simulink model "SimForces2020a"  (R2020a)
settings: Solver=daessc  StartTime=0.0  StopTime=10  FixedStep=0.001  RelTol=1e-4
values from neighbouring files (symbols this model uses):
  Bc1_V = [0;0;0;0;0;0]    [initializeSimulationGP.m]
  D22F = [0;0;0;0;0;0]    [initializeSimulationGP.m]
  filtDV = init2ndOrderLowPassFilter(35*2*pi,1,controller.dT)    [initializeLowPassFilters.m]
  filtEnc = init2ndOrderLowPassFilter(35*2*pi,1,controller.dT)    [initializeLowPassFilters.m]
undefined symbols (not defined in the file or in its folder): aux, B11_r_B11Tc1, B11_V, B11Ftot, B12_r_B12Tc2, B12_Rot_Tc2, B12_U_Tc2, B12_V, B12Ftot, B31_r_B31B41, B31_V, B31FTot, B32_r_B32B42, B32_Rot_B42, B32_U_B42, B32_V, B32FTot, B41_r_B41Tc1, B41_V, B41FTot, B42_r_B42Tc2, B42_Rot_Tc2, B42_U_Tc2, B42_V, B42FTot, B52_r_B52P32, B52_Rot_P32, B52_U_P32, B52_V, B52Ftot, Bc1_r_Bc1B11, Bc1_r_Bc1B31, Bc1FTot, Bc2_r_Bc2B12, Bc2_r_Bc2B32, Bc2_Rot_B12, Bc2_Rot_B32, Bc2_U_B12, Bc2_U_B32, Bc2_V, Bc2Tot, cmdMotion, controller, cyl1, cyl2, D22_V, dq1, dq11, dq12, dq2, dq21, dq22, dx1, dx2, dxt2, fc1, fc1r, fc2, fc2r, fct2 ... (+62)
libraries: sm_lib x31, nesl_utility x10
(part 5 of 7)

== system SimForces2020a/sbVDCController/sbFormTotalRequiredForces/sbTotalRequiredForcesPS2/sbFilteredVelocityDerivativeP32/sbLowPassFilter4 ==
  dV : Inport
  Delay : Delay  InitialConditionSource=Input port  SampleTime=filtDV.dT
      settings: InputPortMap=u0,p4
  Delay1 : Delay  DelayLength=1  InitialConditionSource=Input port  SampleTime=filtDV.dT
      settings: InputPortMap=u0,p4
  Delay2 : Delay  DelayLength=0  InitialConditionSource=Input port  SampleTime=filtDV.dT
      settings: InputPortMap=u0,p4
  Delay3 : Delay  InitialConditionSource=Input port  SampleTime=filtDV.dT
      settings: InputPortMap=u0,p4
  Delay4 : Delay  DelayLength=1  InitialConditionSource=Input port  SampleTime=filtDV.dT
      settings: InputPortMap=u0,p4
  Gain : Gain  Gain=filtDV.a0
  Gain1 : Gain  Gain=filtDV.b1
  Gain2 : Gain  Gain=filtDV.b2
  Gain3 : Gain  Gain=filtDV.b0
  Gain4 : Gain  Gain=filtDV.a1
  Sum : Sum  Inputs=|--+++
  dVFilt : Outport
  wires:
  Delay3/1 -> Gain3/1
  Gain/1 -> Sum/2
  Gain1/1 -> Sum/4
  dV/1 -> Delay/2, Delay4/2, Delay1/2, Delay3/1, Delay3/2, Delay1/1, Delay2/2, Delay2/1  "dV"
  Sum/1 -> Delay/1, Delay4/1, dVFilt/1  "dVFilt"
  Gain4/1 -> Sum/1
  Delay2/1 -> Gain2/1
  Delay1/1 -> Gain1/1
  Delay/1 -> Gain/1
  Delay4/1 -> Gain4/1
  Gain2/1 -> Sum/3
  Gain3/1 -> Sum/5

== system SimForces2020a/sbVDCController/sbFormTotalRequiredForces/sbTotalRequiredForcesPS2/sbFilteredVelocityDerivativeP32/sbLowPassFilter5 ==
  dV : Inport
  Delay : Delay  InitialConditionSource=Input port  SampleTime=filtDV.dT
      settings: InputPortMap=u0,p4
  Delay1 : Delay  DelayLength=1  InitialConditionSource=Input port  SampleTime=filtDV.dT
      settings: InputPortMap=u0,p4
  Delay2 : Delay  DelayLength=0  InitialConditionSource=Input port  SampleTime=filtDV.dT
      settings: InputPortMap=u0,p4
  Delay3 : Delay  InitialConditionSource=Input port  SampleTime=filtDV.dT
      settings: InputPortMap=u0,p4
  Delay4 : Delay  DelayLength=1  InitialConditionSource=Input port  SampleTime=filtDV.dT
      settings: InputPortMap=u0,p4
  Gain : Gain  Gain=filtDV.a0
  Gain1 : Gain  Gain=filtDV.b1
  Gain2 : Gain  Gain=filtDV.b2
  Gain3 : Gain  Gain=filtDV.b0
  Gain4 : Gain  Gain=filtDV.a1
  Sum : Sum  Inputs=|--+++
  dVFilt : Outport
  wires:
  Gain3/1 -> Sum/5
  Gain2/1 -> Sum/3
  Delay4/1 -> Gain4/1
  Delay/1 -> Gain/1
  Delay1/1 -> Gain1/1
  Delay2/1 -> Gain2/1
  Gain4/1 -> Sum/1
  Sum/1 -> dVFilt/1, Delay4/1, Delay/1  "dVFilt"
  dV/1 -> Delay2/1, Delay2/2, Delay1/1, Delay3/2, Delay3/1, Delay1/2, Delay4/2, Delay/2  "dV"
  Gain1/1 -> Sum/4
  Gain/1 -> Sum/2
  Delay3/1 -> Gain3/1

== system SimForces2020a/sbVDCController/sbFormTotalRequiredForces/sbTotalRequiredForcesPS2/sbFilteredVelocityDerivativeP32/sbLowPassFilter6 ==
  dV : Inport
  Delay : Delay  InitialConditionSource=Input port  SampleTime=filtDV.dT
      settings: InputPortMap=u0,p4
  Delay1 : Delay  DelayLength=1  InitialConditionSource=Input port  SampleTime=filtDV.dT
      settings: InputPortMap=u0,p4
  Delay2 : Delay  DelayLength=0  InitialConditionSource=Input port  SampleTime=filtDV.dT
      settings: InputPortMap=u0,p4
  Delay3 : Delay  InitialConditionSource=Input port  SampleTime=filtDV.dT
      settings: InputPortMap=u0,p4
  Delay4 : Delay  DelayLength=1  InitialConditionSource=Input port  SampleTime=filtDV.dT
      settings: InputPortMap=u0,p4
  Gain : Gain  Gain=filtDV.a0
  Gain1 : Gain  Gain=filtDV.b1
  Gain2 : Gain  Gain=filtDV.b2
  Gain3 : Gain  Gain=filtDV.b0
  Gain4 : Gain  Gain=filtDV.a1
  Sum : Sum  Inputs=|--+++
  dVFilt : Outport
  wires:
  Delay3/1 -> Gain3/1
  Gain/1 -> Sum/2
  Gain1/1 -> Sum/4
  dV/1 -> Delay/2, Delay4/2, Delay1/2, Delay3/1, Delay3/2, Delay1/1, Delay2/2, Delay2/1  "dV"
  Sum/1 -> Delay/1, Delay4/1, dVFilt/1  "dVFilt"
  Gain4/1 -> Sum/1
  Delay2/1 -> Gain2/1
  Delay1/1 -> Gain1/1
  Delay/1 -> Gain/1
  Delay4/1 -> Gain4/1
  Gain2/1 -> Sum/3
  Gain3/1 -> Sum/5

== system SimForces2020a/sbVDCController/sbFormTotalRequiredForces/sbTotalRequiredForcesRS1/sbFilteredVelocityDerivativeB11/sbDiscreteDerivative1 ==
  u : Inport
  Add : Sum  Inputs=-+
  Gain6 : Gain  Gain=1/(2*controller.dT)
  Integer Delay : Delay  InitialConditionSource=Input port  InitialCondition=0  SampleTime=controller.dT
      settings: InputPortMap=u0,p4
  du/dt : Outport  PortDimensions=1
  wires:
  Gain6/1 -> du/dt/1
  Integer Delay/1 -> Add/1
  u/1 -> Add/2, Integer Delay/2, Integer Delay/1
  Add/1 -> Gain6/1

== system SimForces2020a/sbVDCController/sbFormTotalRequiredForces/sbTotalRequiredForcesRS1/sbFilteredVelocityDerivativeB11/sbDiscreteDerivative2 ==
  u : Inport
  Add : Sum  Inputs=-+
  Gain6 : Gain  Gain=1/(2*controller.dT)
  Integer Delay : Delay  InitialConditionSource=Input port  InitialCondition=0  SampleTime=controller.dT
      settings: InputPortMap=u0,p4
  du/dt : Outport  PortDimensions=1
  wires:
  Gain6/1 -> du/dt/1
  Add/1 -> Gain6/1
  Integer Delay/1 -> Add/1
  u/1 -> Add/2, Integer Delay/2, Integer Delay/1

== system SimForces2020a/sbVDCController/sbFormTotalRequiredForces/sbTotalRequiredForcesRS1/sbFilteredVelocityDerivativeB11/sbDiscreteDerivative3 ==
  u : Inport
  Add : Sum  Inputs=-+
  Gain6 : Gain  Gain=1/(2*controller.dT)
  Integer Delay : Delay  InitialConditionSource=Input port  InitialCondition=0  SampleTime=controller.dT
      settings: InputPortMap=u0,p4
  du/dt : Outport  PortDimensions=1
  wires:
  Gain6/1 -> du/dt/1
  u/1 -> Add/2, Integer Delay/2, Integer Delay/1
  Integer Delay/1 -> Add/1
  Add/1 -> Gain6/1

== system SimForces2020a/sbVDCController/sbFormTotalRequiredForces/sbTotalRequiredForcesRS1/sbFilteredVelocityDerivativeB11/sbDiscreteDerivative4 ==
  u : Inport
  Add : Sum  Inputs=-+
  Gain6 : Gain  Gain=1/(2*controller.dT)
  Integer Delay : Delay  InitialConditionSource=Input port  InitialCondition=0  SampleTime=controller.dT
      settings: InputPortMap=u0,p4
  du/dt : Outport  PortDimensions=1
  wires:
  Gain6/1 -> du/dt/1
  u/1 -> Add/2, Integer Delay/2, Integer Delay/1
  Integer Delay/1 -> Add/1
  Add/1 -> Gain6/1

== system SimForces2020a/sbVDCController/sbFormTotalRequiredForces/sbTotalRequiredForcesRS1/sbFilteredVelocityDerivativeB11/sbDiscreteDerivative5 ==
  u : Inport
  Add : Sum  Inputs=-+
  Gain6 : Gain  Gain=1/(2*controller.dT)
  Integer Delay : Delay  InitialConditionSource=Input port  InitialCondition=0  SampleTime=controller.dT
      settings: InputPortMap=u0,p4
  du/dt : Outport  PortDimensions=1
  wires:
  Gain6/1 -> du/dt/1
  u/1 -> Add/2, Integer Delay/2, Integer Delay/1
  Integer Delay/1 -> Add/1
  Add/1 -> Gain6/1

== system SimForces2020a/sbVDCController/sbFormTotalRequiredForces/sbTotalRequiredForcesRS1/sbFilteredVelocityDerivativeB11/sbDiscreteDerivative6 ==
  u : Inport
  Add : Sum  Inputs=-+
  Gain6 : Gain  Gain=1/(2*controller.dT)
  Integer Delay : Delay  InitialConditionSource=Input port  InitialCondition=0  SampleTime=controller.dT
      settings: InputPortMap=u0,p4
  du/dt : Outport  PortDimensions=1
  wires:
  Gain6/1 -> du/dt/1
  u/1 -> Add/2, Integer Delay/2, Integer Delay/1
  Integer Delay/1 -> Add/1
  Add/1 -> Gain6/1

== system SimForces2020a/sbVDCController/sbFormTotalRequiredForces/sbTotalRequiredForcesRS1/sbFilteredVelocityDerivativeB11/sbLowPassFilter1 ==
  dV : Inport
  Delay : Delay  InitialConditionSource=Input port  SampleTime=filtDV.dT
      settings: InputPortMap=u0,p4
  Delay1 : Delay  DelayLength=1  InitialConditionSource=Input port  SampleTime=filtDV.dT
      settings: InputPortMap=u0,p4
  Delay2 : Delay  DelayLength=0  InitialConditionSource=Input port  SampleTime=filtDV.dT
      settings: InputPortMap=u0,p4
  Delay3 : Delay  InitialConditionSource=Input port  SampleTime=filtDV.dT
      settings: InputPortMap=u0,p4
  Delay4 : Delay  DelayLength=1  InitialConditionSource=Input port  SampleTime=filtDV.dT
      settings: InputPortMap=u0,p4
  Gain : Gain  Gain=filtDV.a0
  Gain1 : Gain  Gain=filtDV.b1
  Gain2 : Gain  Gain=filtDV.b2
  Gain3 : Gain  Gain=filtDV.b0
  Gain4 : Gain  Gain=filtDV.a1
  Sum : Sum  Inputs=|--+++
  dVFilt : Outport
  wires:
  Delay3/1 -> Gain3/1
  Gain/1 -> Sum/2
  Gain1/1 -> Sum/4
  dV/1 -> Delay/2, Delay4/2, Delay1/2, Delay3/1, Delay3/2, Delay1/1, Delay2/2, Delay2/1  "dV"
  Sum/1 -> Delay/1, Delay4/1, dVFilt/1  "dVFilt"
  Gain4/1 -> Sum/1
  Delay2/1 -> Gain2/1
  Delay1/1 -> Gain1/1
  Delay/1 -> Gain/1
  Delay4/1 -> Gain4/1
  Gain2/1 -> Sum/3
  Gain3/1 -> Sum/5

== system SimForces2020a/sbVDCController/sbFormTotalRequiredForces/sbTotalRequiredForcesRS1/sbFilteredVelocityDerivativeB11/sbLowPassFilter2 ==
  dV : Inport
  Delay : Delay  InitialConditionSource=Input port  SampleTime=filtDV.dT
      settings: InputPortMap=u0,p4
  Delay1 : Delay  DelayLength=1  InitialConditionSource=Input port  SampleTime=filtDV.dT
      settings: InputPortMap=u0,p4
  Delay2 : Delay  DelayLength=0  InitialConditionSource=Input port  SampleTime=filtDV.dT
      settings: InputPortMap=u0,p4
  Delay3 : Delay  InitialConditionSource=Input port  SampleTime=filtDV.dT
      settings: InputPortMap=u0,p4
  Delay4 : Delay  DelayLength=1  InitialConditionSource=Input port  SampleTime=filtDV.dT
      settings: InputPortMap=u0,p4
  Gain : Gain  Gain=filtDV.a0
  Gain1 : Gain  Gain=filtDV.b1
  Gain2 : Gain  Gain=filtDV.b2
  Gain3 : Gain  Gain=filtDV.b0
  Gain4 : Gain  Gain=filtDV.a1
  Sum : Sum  Inputs=|--+++
  dVFilt : Outport
  wires:
  Gain3/1 -> Sum/5
  Gain2/1 -> Sum/3
  Delay4/1 -> Gain4/1
  Delay/1 -> Gain/1
  Delay1/1 -> Gain1/1
  Delay2/1 -> Gain2/1
  Gain4/1 -> Sum/1
  Sum/1 -> dVFilt/1, Delay4/1, Delay/1  "dVFilt"
  dV/1 -> Delay2/1, Delay2/2, Delay1/1, Delay3/2, Delay3/1, Delay1/2, Delay4/2, Delay/2  "dV"
  Gain1/1 -> Sum/4
  Gain/1 -> Sum/2
  Delay3/1 -> Gain3/1

== system SimForces2020a/sbVDCController/sbFormTotalRequiredForces/sbTotalRequiredForcesRS1/sbFilteredVelocityDerivativeB11/sbLowPassFilter3 ==
  dV : Inport
  Delay : Delay  InitialConditionSource=Input port  SampleTime=filtDV.dT
      settings: InputPortMap=u0,p4
  Delay1 : Delay  DelayLength=1  InitialConditionSource=Input port  SampleTime=filtDV.dT
      settings: InputPortMap=u0,p4
  Delay2 : Delay  DelayLength=0  InitialConditionSource=Input port  SampleTime=filtDV.dT
      settings: InputPortMap=u0,p4
  Delay3 : Delay  InitialConditionSource=Input port  SampleTime=filtDV.dT
      settings: InputPortMap=u0,p4
  Delay4 : Delay  DelayLength=1  InitialConditionSource=Input port  SampleTime=filtDV.dT
      settings: InputPortMap=u0,p4
  Gain : Gain  Gain=filtDV.a0
  Gain1 : Gain  Gain=filtDV.b1
  Gain2 : Gain  Gain=filtDV.b2
  Gain3 : Gain  Gain=filtDV.b0
  Gain4 : Gain  Gain=filtDV.a1
  Sum : Sum  Inputs=|--+++
  dVFilt : Outport
  wires:
  Delay3/1 -> Gain3/1
  Gain/1 -> Sum/2
  Gain1/1 -> Sum/4
  dV/1 -> Delay/2, Delay4/2, Delay1/2, Delay3/1, Delay3/2, Delay1/1, Delay2/2, Delay2/1  "dV"
  Sum/1 -> Delay/1, Delay4/1, dVFilt/1  "dVFilt"
  Gain4/1 -> Sum/1
  Delay2/1 -> Gain2/1
  Delay1/1 -> Gain1/1
  Delay/1 -> Gain/1
  Delay4/1 -> Gain4/1
  Gain2/1 -> Sum/3
  Gain3/1 -> Sum/5

== system SimForces2020a/sbVDCController/sbFormTotalRequiredForces/sbTotalRequiredForcesRS1/sbFilteredVelocityDerivativeB11/sbLowPassFilter4 ==
  dV : Inport
  Delay : Delay  InitialConditionSource=Input port  SampleTime=filtDV.dT
      settings: InputPortMap=u0,p4
  Delay1 : Delay  DelayLength=1  InitialConditionSource=Input port  SampleTime=filtDV.dT
      settings: InputPortMap=u0,p4
  Delay2 : Delay  DelayLength=0  InitialConditionSource=Input port  SampleTime=filtDV.dT
      settings: InputPortMap=u0,p4
  Delay3 : Delay  InitialConditionSource=Input port  SampleTime=filtDV.dT
      settings: InputPortMap=u0,p4
  Delay4 : Delay  DelayLength=1  InitialConditionSource=Input port  SampleTime=filtDV.dT
      settings: InputPortMap=u0,p4
  Gain : Gain  Gain=filtDV.a0
  Gain1 : Gain  Gain=filtDV.b1
  Gain2 : Gain  Gain=filtDV.b2
  Gain3 : Gain  Gain=filtDV.b0
  Gain4 : Gain  Gain=filtDV.a1
  Sum : Sum  Inputs=|--+++
  dVFilt : Outport
  wires:
  Gain3/1 -> Sum/5
  Gain2/1 -> Sum/3
  Delay4/1 -> Gain4/1
  Delay/1 -> Gain/1
  Delay1/1 -> Gain1/1
  Delay2/1 -> Gain2/1
  Gain4/1 -> Sum/1
  Sum/1 -> dVFilt/1, Delay4/1, Delay/1  "dVFilt"
  dV/1 -> Delay2/1, Delay2/2, Delay1/1, Delay3/2, Delay3/1, Delay1/2, Delay4/2, Delay/2  "dV"
  Gain1/1 -> Sum/4
  Gain/1 -> Sum/2
  Delay3/1 -> Gain3/1

== system SimForces2020a/sbVDCController/sbFormTotalRequiredForces/sbTotalRequiredForcesRS1/sbFilteredVelocityDerivativeB11/sbLowPassFilter5 ==
  dV : Inport
  Delay : Delay  InitialConditionSource=Input port  SampleTime=filtDV.dT
      settings: InputPortMap=u0,p4
  Delay1 : Delay  DelayLength=1  InitialConditionSource=Input port  SampleTime=filtDV.dT
      settings: InputPortMap=u0,p4
  Delay2 : Delay  DelayLength=0  InitialConditionSource=Input port  SampleTime=filtDV.dT
      settings: InputPortMap=u0,p4
  Delay3 : Delay  InitialConditionSource=Input port  SampleTime=filtDV.dT
      settings: InputPortMap=u0,p4
  Delay4 : Delay  DelayLength=1  InitialConditionSource=Input port  SampleTime=filtDV.dT
      settings: InputPortMap=u0,p4
  Gain : Gain  Gain=filtDV.a0
  Gain1 : Gain  Gain=filtDV.b1
  Gain2 : Gain  Gain=filtDV.b2
  Gain3 : Gain  Gain=filtDV.b0
  Gain4 : Gain  Gain=filtDV.a1
  Sum : Sum  Inputs=|--+++
  dVFilt : Outport
  wires:
  Delay3/1 -> Gain3/1
  Gain/1 -> Sum/2
  Gain1/1 -> Sum/4
  dV/1 -> Delay/2, Delay4/2, Delay1/2, Delay3/1, Delay3/2, Delay1/1, Delay2/2, Delay2/1  "dV"
  Sum/1 -> Delay/1, Delay4/1, dVFilt/1  "dVFilt"
  Gain4/1 -> Sum/1
  Delay2/1 -> Gain2/1
  Delay1/1 -> Gain1/1
  Delay/1 -> Gain/1
  Delay4/1 -> Gain4/1
  Gain2/1 -> Sum/3
  Gain3/1 -> Sum/5

== system SimForces2020a/sbVDCController/sbFormTotalRequiredForces/sbTotalRequiredForcesRS1/sbFilteredVelocityDerivativeB11/sbLowPassFilter6 ==
  dV : Inport
  Delay : Delay  InitialConditionSource=Input port  SampleTime=filtDV.dT
      settings: InputPortMap=u0,p4
  Delay1 : Delay  DelayLength=1  InitialConditionSource=Input port  SampleTime=filtDV.dT
      settings: InputPortMap=u0,p4
  Delay2 : Delay  DelayLength=0  InitialConditionSource=Input port  SampleTime=filtDV.dT
      settings: InputPortMap=u0,p4
  Delay3 : Delay  InitialConditionSource=Input port  SampleTime=filtDV.dT
      settings: InputPortMap=u0,p4
  Delay4 : Delay  DelayLength=1  InitialConditionSource=Input port  SampleTime=filtDV.dT
      settings: InputPortMap=u0,p4
  Gain : Gain  Gain=filtDV.a0
  Gain1 : Gain  Gain=filtDV.b1
  Gain2 : Gain  Gain=filtDV.b2
  Gain3 : Gain  Gain=filtDV.b0
  Gain4 : Gain  Gain=filtDV.a1
  Sum : Sum  Inputs=|--+++
  dVFilt : Outport
  wires:
  Gain3/1 -> Sum/5
  Gain2/1 -> Sum/3
  Delay4/1 -> Gain4/1
  Delay/1 -> Gain/1
  Delay1/1 -> Gain1/1
  Delay2/1 -> Gain2/1
  Gain4/1 -> Sum/1
  Sum/1 -> dVFilt/1, Delay4/1, Delay/1  "dVFilt"
  dV/1 -> Delay2/1, Delay2/2, Delay1/1, Delay3/2, Delay3/1, Delay1/2, Delay4/2, Delay/2  "dV"
  Gain1/1 -> Sum/4
  Gain/1 -> Sum/2
  Delay3/1 -> Gain3/1

== system SimForces2020a/sbVDCController/sbFormTotalRequiredForces/sbTotalRequiredForcesRS1/sbFilteredVelocityDerivativeB31/sbDiscreteDerivative1 ==
  u : Inport
  Add : Sum  Inputs=-+
  Gain6 : Gain  Gain=1/(2*controller.dT)
  Integer Delay : Delay  InitialConditionSource=Input port  InitialCondition=0  SampleTime=controller.dT
      settings: InputPortMap=u0,p4
  du/dt : Outport  PortDimensions=1
  wires:
  Add/1 -> Gain6/1
  u/1 -> Integer Delay/1, Integer Delay/2, Add/2
  Integer Delay/1 -> Add/1
  Gain6/1 -> du/dt/1

== system SimForces2020a/sbVDCController/sbFormTotalRequiredForces/sbTotalRequiredForcesRS1/sbFilteredVelocityDerivativeB31/sbDiscreteDerivative2 ==
  u : Inport
  Add : Sum  Inputs=-+
  Gain6 : Gain  Gain=1/(2*controller.dT)
  Integer Delay : Delay  InitialConditionSource=Input port  InitialCondition=0  SampleTime=controller.dT
      settings: InputPortMap=u0,p4
  du/dt : Outport  PortDimensions=1
  wires:
  u/1 -> Integer Delay/1, Integer Delay/2, Add/2
  Integer Delay/1 -> Add/1
  Add/1 -> Gain6/1
  Gain6/1 -> du/dt/1

== system SimForces2020a/sbVDCController/sbFormTotalRequiredForces/sbTotalRequiredForcesRS1/sbFilteredVelocityDerivativeB31/sbDiscreteDerivative3 ==
  u : Inport
  Add : Sum  Inputs=-+
  Gain6 : Gain  Gain=1/(2*controller.dT)
  Integer Delay : Delay  InitialConditionSource=Input port  InitialCondition=0  SampleTime=controller.dT
      settings: InputPortMap=u0,p4
  du/dt : Outport  PortDimensions=1
  wires:
  Add/1 -> Gain6/1
  Integer Delay/1 -> Add/1
  u/1 -> Integer Delay/1, Integer Delay/2, Add/2
  Gain6/1 -> du/dt/1

== system SimForces2020a/sbVDCController/sbFormTotalRequiredForces/sbTotalRequiredForcesRS1/sbFilteredVelocityDerivativeB31/sbDiscreteDerivative4 ==
  u : Inport
  Add : Sum  Inputs=-+
  Gain6 : Gain  Gain=1/(2*controller.dT)
  Integer Delay : Delay  InitialConditionSource=Input port  InitialCondition=0  SampleTime=controller.dT
      settings: InputPortMap=u0,p4
  du/dt : Outport  PortDimensions=1
  wires:
  Add/1 -> Gain6/1
  Integer Delay/1 -> Add/1
  u/1 -> Integer Delay/1, Integer Delay/2, Add/2
  Gain6/1 -> du/dt/1

== system SimForces2020a/sbVDCController/sbFormTotalRequiredForces/sbTotalRequiredForcesRS1/sbFilteredVelocityDerivativeB31/sbDiscreteDerivative5 ==
  u : Inport
  Add : Sum  Inputs=-+
  Gain6 : Gain  Gain=1/(2*controller.dT)
  Integer Delay : Delay  InitialConditionSource=Input port  InitialCondition=0  SampleTime=controller.dT
      settings: InputPortMap=u0,p4
  du/dt : Outport  PortDimensions=1
  wires:
  Add/1 -> Gain6/1
  Integer Delay/1 -> Add/1
  u/1 -> Integer Delay/1, Integer Delay/2, Add/2
  Gain6/1 -> du/dt/1

== system SimForces2020a/sbVDCController/sbFormTotalRequiredForces/sbTotalRequiredForcesRS1/sbFilteredVelocityDerivativeB31/sbDiscreteDerivative6 ==
  u : Inport
  Add : Sum  Inputs=-+
  Gain6 : Gain  Gain=1/(2*controller.dT)
  Integer Delay : Delay  InitialConditionSource=Input port  InitialCondition=0  SampleTime=controller.dT
      settings: InputPortMap=u0,p4
  du/dt : Outport  PortDimensions=1
  wires:
  Add/1 -> Gain6/1
  Integer Delay/1 -> Add/1
  u/1 -> Integer Delay/1, Integer Delay/2, Add/2
  Gain6/1 -> du/dt/1

== system SimForces2020a/sbVDCController/sbFormTotalRequiredForces/sbTotalRequiredForcesRS1/sbFilteredVelocityDerivativeB31/sbLowPassFilter1 ==
  dV : Inport
  Delay : Delay  InitialConditionSource=Input port  SampleTime=filtDV.dT
      settings: InputPortMap=u0,p4
  Delay1 : Delay  DelayLength=1  InitialConditionSource=Input port  SampleTime=filtDV.dT
      settings: InputPortMap=u0,p4
  Delay2 : Delay  DelayLength=0  InitialConditionSource=Input port  SampleTime=filtDV.dT
      settings: InputPortMap=u0,p4
  Delay3 : Delay  InitialConditionSource=Input port  SampleTime=filtDV.dT
      settings: InputPortMap=u0,p4
  Delay4 : Delay  DelayLength=1  InitialConditionSource=Input port  SampleTime=filtDV.dT
      settings: InputPortMap=u0,p4
  Gain : Gain  Gain=filtDV.a0
  Gain1 : Gain  Gain=filtDV.b1
  Gain2 : Gain  Gain=filtDV.b2
  Gain3 : Gain  Gain=filtDV.b0
  Gain4 : Gain  Gain=filtDV.a1
  Sum : Sum  Inputs=|--+++
  dVFilt : Outport
  wires:
  Gain3/1 -> Sum/5
  Gain2/1 -> Sum/3
  Delay4/1 -> Gain4/1
  Delay/1 -> Gain/1
  Delay1/1 -> Gain1/1
  Delay2/1 -> Gain2/1
  Gain4/1 -> Sum/1
  Sum/1 -> dVFilt/1, Delay4/1, Delay/1  "dVFilt"
  dV/1 -> Delay2/1, Delay2/2, Delay1/1, Delay3/2, Delay3/1, Delay1/2, Delay4/2, Delay/2  "dV"
  Gain1/1 -> Sum/4
  Gain/1 -> Sum/2
  Delay3/1 -> Gain3/1

== system SimForces2020a/sbVDCController/sbFormTotalRequiredForces/sbTotalRequiredForcesRS1/sbFilteredVelocityDerivativeB31/sbLowPassFilter2 ==
  dV : Inport
  Delay : Delay  InitialConditionSource=Input port  SampleTime=filtDV.dT
      settings: InputPortMap=u0,p4
  Delay1 : Delay  DelayLength=1  InitialConditionSource=Input port  SampleTime=filtDV.dT
      settings: InputPortMap=u0,p4
  Delay2 : Delay  DelayLength=0  InitialConditionSource=Input port  SampleTime=filtDV.dT
      settings: InputPortMap=u0,p4
  Delay3 : Delay  InitialConditionSource=Input port  SampleTime=filtDV.dT
      settings: InputPortMap=u0,p4
  Delay4 : Delay  DelayLength=1  InitialConditionSource=Input port  SampleTime=filtDV.dT
      settings: InputPortMap=u0,p4
  Gain : Gain  Gain=filtDV.a0
  Gain1 : Gain  Gain=filtDV.b1
  Gain2 : Gain  Gain=filtDV.b2
  Gain3 : Gain  Gain=filtDV.b0
  Gain4 : Gain  Gain=filtDV.a1
  Sum : Sum  Inputs=|--+++
  dVFilt : Outport
  wires:
  Delay3/1 -> Gain3/1
  Gain/1 -> Sum/2
  Gain1/1 -> Sum/4
  dV/1 -> Delay/2, Delay4/2, Delay1/2, Delay3/1, Delay3/2, Delay1/1, Delay2/2, Delay2/1  "dV"
  Sum/1 -> Delay/1, Delay4/1, dVFilt/1  "dVFilt"
  Gain4/1 -> Sum/1
  Delay2/1 -> Gain2/1
  Delay1/1 -> Gain1/1
  Delay/1 -> Gain/1
  Delay4/1 -> Gain4/1
  Gain2/1 -> Sum/3
  Gain3/1 -> Sum/5

== system SimForces2020a/sbVDCController/sbFormTotalRequiredForces/sbTotalRequiredForcesRS1/sbFilteredVelocityDerivativeB31/sbLowPassFilter3 ==
  dV : Inport
  Delay : Delay  InitialConditionSource=Input port  SampleTime=filtDV.dT
      settings: InputPortMap=u0,p4
  Delay1 : Delay  DelayLength=1  InitialConditionSource=Input port  SampleTime=filtDV.dT
      settings: InputPortMap=u0,p4
  Delay2 : Delay  DelayLength=0  InitialConditionSource=Input port  SampleTime=filtDV.dT
      settings: InputPortMap=u0,p4
  Delay3 : Delay  InitialConditionSource=Input port  SampleTime=filtDV.dT
      settings: InputPortMap=u0,p4
  Delay4 : Delay  DelayLength=1  InitialConditionSource=Input port  SampleTime=filtDV.dT
      settings: InputPortMap=u0,p4
  Gain : Gain  Gain=filtDV.a0
  Gain1 : Gain  Gain=filtDV.b1
  Gain2 : Gain  Gain=filtDV.b2
  Gain3 : Gain  Gain=filtDV.b0
  Gain4 : Gain  Gain=filtDV.a1
  Sum : Sum  Inputs=|--+++
  dVFilt : Outport
  wires:
  Gain3/1 -> Sum/5
  Gain2/1 -> Sum/3
  Delay4/1 -> Gain4/1
  Delay/1 -> Gain/1
  Delay1/1 -> Gain1/1
  Delay2/1 -> Gain2/1
  Gain4/1 -> Sum/1
  Sum/1 -> dVFilt/1, Delay4/1, Delay/1  "dVFilt"
  dV/1 -> Delay2/1, Delay2/2, Delay1/1, Delay3/2, Delay3/1, Delay1/2, Delay4/2, Delay/2  "dV"
  Gain1/1 -> Sum/4
  Gain/1 -> Sum/2
  Delay3/1 -> Gain3/1

== system SimForces2020a/sbVDCController/sbFormTotalRequiredForces/sbTotalRequiredForcesRS1/sbFilteredVelocityDerivativeB31/sbLowPassFilter4 ==
  dV : Inport
  Delay : Delay  InitialConditionSource=Input port  SampleTime=filtDV.dT
      settings: InputPortMap=u0,p4
  Delay1 : Delay  DelayLength=1  InitialConditionSource=Input port  SampleTime=filtDV.dT
      settings: InputPortMap=u0,p4
  Delay2 : Delay  DelayLength=0  InitialConditionSource=Input port  SampleTime=filtDV.dT
      settings: InputPortMap=u0,p4
  Delay3 : Delay  InitialConditionSource=Input port  SampleTime=filtDV.dT
      settings: InputPortMap=u0,p4
  Delay4 : Delay  DelayLength=1  InitialConditionSource=Input port  SampleTime=filtDV.dT
      settings: InputPortMap=u0,p4
  Gain : Gain  Gain=filtDV.a0
  Gain1 : Gain  Gain=filtDV.b1
  Gain2 : Gain  Gain=filtDV.b2
  Gain3 : Gain  Gain=filtDV.b0
  Gain4 : Gain  Gain=filtDV.a1
  Sum : Sum  Inputs=|--+++
  dVFilt : Outport
  wires:
  Delay3/1 -> Gain3/1
  Gain/1 -> Sum/2
  Gain1/1 -> Sum/4
  dV/1 -> Delay/2, Delay4/2, Delay1/2, Delay3/1, Delay3/2, Delay1/1, Delay2/2, Delay2/1  "dV"
  Sum/1 -> Delay/1, Delay4/1, dVFilt/1  "dVFilt"
  Gain4/1 -> Sum/1
  Delay2/1 -> Gain2/1
  Delay1/1 -> Gain1/1
  Delay/1 -> Gain/1
  Delay4/1 -> Gain4/1
  Gain2/1 -> Sum/3
  Gain3/1 -> Sum/5

== system SimForces2020a/sbVDCController/sbFormTotalRequiredForces/sbTotalRequiredForcesRS1/sbFilteredVelocityDerivativeB31/sbLowPassFilter5 ==
  dV : Inport
  Delay : Delay  InitialConditionSource=Input port  SampleTime=filtDV.dT
      settings: InputPortMap=u0,p4
  Delay1 : Delay  DelayLength=1  InitialConditionSource=Input port  SampleTime=filtDV.dT
      settings: InputPortMap=u0,p4
  Delay2 : Delay  DelayLength=0  InitialConditionSource=Input port  SampleTime=filtDV.dT
      settings: InputPortMap=u0,p4
  Delay3 : Delay  InitialConditionSource=Input port  SampleTime=filtDV.dT
      settings: InputPortMap=u0,p4
  Delay4 : Delay  DelayLength=1  InitialConditionSource=Input port  SampleTime=filtDV.dT
      settings: InputPortMap=u0,p4
  Gain : Gain  Gain=filtDV.a0
  Gain1 : Gain  Gain=filtDV.b1
  Gain2 : Gain  Gain=filtDV.b2
  Gain3 : Gain  Gain=filtDV.b0
  Gain4 : Gain  Gain=filtDV.a1
  Sum : Sum  Inputs=|--+++
  dVFilt : Outport
  wires:
  Gain3/1 -> Sum/5
  Gain2/1 -> Sum/3
  Delay4/1 -> Gain4/1
  Delay/1 -> Gain/1
  Delay1/1 -> Gain1/1
  Delay2/1 -> Gain2/1
  Gain4/1 -> Sum/1
  Sum/1 -> dVFilt/1, Delay4/1, Delay/1  "dVFilt"
  dV/1 -> Delay2/1, Delay2/2, Delay1/1, Delay3/2, Delay3/1, Delay1/2, Delay4/2, Delay/2  "dV"
  Gain1/1 -> Sum/4
  Gain/1 -> Sum/2
  Delay3/1 -> Gain3/1

== system SimForces2020a/sbVDCController/sbFormTotalRequiredForces/sbTotalRequiredForcesRS1/sbFilteredVelocityDerivativeB31/sbLowPassFilter6 ==
  dV : Inport
  Delay : Delay  InitialConditionSource=Input port  SampleTime=filtDV.dT
      settings: InputPortMap=u0,p4
  Delay1 : Delay  DelayLength=1  InitialConditionSource=Input port  SampleTime=filtDV.dT
      settings: InputPortMap=u0,p4
  Delay2 : Delay  DelayLength=0  InitialConditionSource=Input port  SampleTime=filtDV.dT
      settings: InputPortMap=u0,p4
  Delay3 : Delay  InitialConditionSource=Input port  SampleTime=filtDV.dT
      settings: InputPortMap=u0,p4
  Delay4 : Delay  DelayLength=1  InitialConditionSource=Input port  SampleTime=filtDV.dT
      settings: InputPortMap=u0,p4
  Gain : Gain  Gain=filtDV.a0
  Gain1 : Gain  Gain=filtDV.b1
  Gain2 : Gain  Gain=filtDV.b2
  Gain3 : Gain  Gain=filtDV.b0
  Gain4 : Gain  Gain=filtDV.a1
  Sum : Sum  Inputs=|--+++
  dVFilt : Outport
  wires:
  Delay3/1 -> Gain3/1
  Gain/1 -> Sum/2
  Gain1/1 -> Sum/4
  dV/1 -> Delay/2, Delay4/2, Delay1/2, Delay3/1, Delay3/2, Delay1/1, Delay2/2, Delay2/1  "dV"
  Sum/1 -> Delay/1, Delay4/1, dVFilt/1  "dVFilt"
  Gain4/1 -> Sum/1
  Delay2/1 -> Gain2/1
  Delay1/1 -> Gain1/1
  Delay/1 -> Gain/1
  Delay4/1 -> Gain4/1
  Gain2/1 -> Sum/3
  Gain3/1 -> Sum/5

== system SimForces2020a/sbVDCController/sbFormTotalRequiredForces/sbTotalRequiredForcesRS1/sbFilteredVelocityDerivativeB41/sbDiscreteDerivative1 ==
  u : Inport
  Add : Sum  Inputs=-+
  Gain6 : Gain  Gain=1/(2*controller.dT)
  Integer Delay : Delay  InitialConditionSource=Input port  InitialCondition=0  SampleTime=controller.dT
      settings: InputPortMap=u0,p4
  du/dt : Outport  PortDimensions=1
  wires:
  Add/1 -> Gain6/1
  u/1 -> Integer Delay/1, Integer Delay/2, Add/2
  Integer Delay/1 -> Add/1
  Gain6/1 -> du/dt/1

== system SimForces2020a/sbVDCController/sbFormTotalRequiredForces/sbTotalRequiredForcesRS1/sbFilteredVelocityDerivativeB41/sbDiscreteDerivative2 ==
  u : Inport
  Add : Sum  Inputs=-+
  Gain6 : Gain  Gain=1/(2*controller.dT)
  Integer Delay : Delay  InitialConditionSource=Input port  InitialCondition=0  SampleTime=controller.dT
      settings: InputPortMap=u0,p4
  du/dt : Outport  PortDimensions=1
  wires:
  u/1 -> Integer Delay/1, Integer Delay/2, Add/2
  Integer Delay/1 -> Add/1
  Add/1 -> Gain6/1
  Gain6/1 -> du/dt/1

== system SimForces2020a/sbVDCController/sbFormTotalRequiredForces/sbTotalRequiredForcesRS1/sbFilteredVelocityDerivativeB41/sbDiscreteDerivative3 ==
  u : Inport
  Add : Sum  Inputs=-+
  Gain6 : Gain  Gain=1/(2*controller.dT)
  Integer Delay : Delay  InitialConditionSource=Input port  InitialCondition=0  SampleTime=controller.dT
      settings: InputPortMap=u0,p4
  du/dt : Outport  PortDimensions=1
  wires:
  Add/1 -> Gain6/1
  Integer Delay/1 -> Add/1
  u/1 -> Integer Delay/1, Integer Delay/2, Add/2
  Gain6/1 -> du/dt/1

== system SimForces2020a/sbVDCController/sbFormTotalRequiredForces/sbTotalRequiredForcesRS1/sbFilteredVelocityDerivativeB41/sbDiscreteDerivative4 ==
  u : Inport
  Add : Sum  Inputs=-+
  Gain6 : Gain  Gain=1/(2*controller.dT)
  Integer Delay : Delay  InitialConditionSource=Input port  InitialCondition=0  SampleTime=controller.dT
      settings: InputPortMap=u0,p4
  du/dt : Outport  PortDimensions=1
  wires:
  Add/1 -> Gain6/1
  Integer Delay/1 -> Add/1
  u/1 -> Integer Delay/1, Integer Delay/2, Add/2
  Gain6/1 -> du/dt/1

== system SimForces2020a/sbVDCController/sbFormTotalRequiredForces/sbTotalRequiredForcesRS1/sbFilteredVelocityDerivativeB41/sbDiscreteDerivative5 ==
  u : Inport
  Add : Sum  Inputs=-+
  Gain6 : Gain  Gain=1/(2*controller.dT)
  Integer Delay : Delay  InitialConditionSource=Input port  InitialCondition=0  SampleTime=controller.dT
      settings: InputPortMap=u0,p4
  du/dt : Outport  PortDimensions=1
  wires:
  Add/1 -> Gain6/1
  Integer Delay/1 -> Add/1
  u/1 -> Integer Delay/1, Integer Delay/2, Add/2
  Gain6/1 -> du/dt/1

== system SimForces2020a/sbVDCController/sbFormTotalRequiredForces/sbTotalRequiredForcesRS1/sbFilteredVelocityDerivativeB41/sbDiscreteDerivative6 ==
  u : Inport
  Add : Sum  Inputs=-+
  Gain6 : Gain  Gain=1/(2*controller.dT)
  Integer Delay : Delay  InitialConditionSource=Input port  InitialCondition=0  SampleTime=controller.dT
      settings: InputPortMap=u0,p4
  du/dt : Outport  PortDimensions=1
  wires:
  Add/1 -> Gain6/1
  Integer Delay/1 -> Add/1
  u/1 -> Integer Delay/1, Integer Delay/2, Add/2
  Gain6/1 -> du/dt/1

== system SimForces2020a/sbVDCController/sbFormTotalRequiredForces/sbTotalRequiredForcesRS1/sbFilteredVelocityDerivativeB41/sbLowPassFilter1 ==
  dV : Inport
  Delay : Delay  InitialConditionSource=Input port  SampleTime=filtDV.dT
      settings: InputPortMap=u0,p4
  Delay1 : Delay  DelayLength=1  InitialConditionSource=Input port  SampleTime=filtDV.dT
      settings: InputPortMap=u0,p4
  Delay2 : Delay  DelayLength=0  InitialConditionSource=Input port  SampleTime=filtDV.dT
      settings: InputPortMap=u0,p4
  Delay3 : Delay  InitialConditionSource=Input port  SampleTime=filtDV.dT
      settings: InputPortMap=u0,p4
  Delay4 : Delay  DelayLength=1  InitialConditionSource=Input port  SampleTime=filtDV.dT
      settings: InputPortMap=u0,p4
  Gain : Gain  Gain=filtDV.a0
  Gain1 : Gain  Gain=filtDV.b1
  Gain2 : Gain  Gain=filtDV.b2
  Gain3 : Gain  Gain=filtDV.b0
  Gain4 : Gain  Gain=filtDV.a1
  Sum : Sum  Inputs=|--+++
  dVFilt : Outport
  wires:
  Gain3/1 -> Sum/5
  Gain2/1 -> Sum/3
  Delay4/1 -> Gain4/1
  Delay/1 -> Gain/1
  Delay1/1 -> Gain1/1
  Delay2/1 -> Gain2/1
  Gain4/1 -> Sum/1
  Sum/1 -> dVFilt/1, Delay4/1, Delay/1  "dVFilt"
  dV/1 -> Delay2/1, Delay2/2, Delay1/1, Delay3/2, Delay3/1, Delay1/2, Delay4/2, Delay/2  "dV"
  Gain1/1 -> Sum/4
  Gain/1 -> Sum/2
  Delay3/1 -> Gain3/1

== system SimForces2020a/sbVDCController/sbFormTotalRequiredForces/sbTotalRequiredForcesRS1/sbFilteredVelocityDerivativeB41/sbLowPassFilter2 ==
  dV : Inport
  Delay : Delay  InitialConditionSource=Input port  SampleTime=filtDV.dT
      settings: InputPortMap=u0,p4
  Delay1 : Delay  DelayLength=1  InitialConditionSource=Input port  SampleTime=filtDV.dT
      settings: InputPortMap=u0,p4
  Delay2 : Delay  DelayLength=0  InitialConditionSource=Input port  SampleTime=filtDV.dT
      settings: InputPortMap=u0,p4
  Delay3 : Delay  InitialConditionSource=Input port  SampleTime=filtDV.dT
      settings: InputPortMap=u0,p4
  Delay4 : Delay  DelayLength=1  InitialConditionSource=Input port  SampleTime=filtDV.dT
      settings: InputPortMap=u0,p4
  Gain : Gain  Gain=filtDV.a0
  Gain1 : Gain  Gain=filtDV.b1
  Gain2 : Gain  Gain=filtDV.b2
  Gain3 : Gain  Gain=filtDV.b0
  Gain4 : Gain  Gain=filtDV.a1
  Sum : Sum  Inputs=|--+++
  dVFilt : Outport
  wires:
  Delay3/1 -> Gain3/1
  Gain/1 -> Sum/2
  Gain1/1 -> Sum/4
  dV/1 -> Delay/2, Delay4/2, Delay1/2, Delay3/1, Delay3/2, Delay1/1, Delay2/2, Delay2/1  "dV"
  Sum/1 -> Delay/1, Delay4/1, dVFilt/1  "dVFilt"
  Gain4/1 -> Sum/1
  Delay2/1 -> Gain2/1
  Delay1/1 -> Gain1/1
  Delay/1 -> Gain/1
  Delay4/1 -> Gain4/1
  Gain2/1 -> Sum/3
  Gain3/1 -> Sum/5

== system SimForces2020a/sbVDCController/sbFormTotalRequiredForces/sbTotalRequiredForcesRS1/sbFilteredVelocityDerivativeB41/sbLowPassFilter3 ==
  dV : Inport
  Delay : Delay  InitialConditionSource=Input port  SampleTime=filtDV.dT
      settings: InputPortMap=u0,p4
  Delay1 : Delay  DelayLength=1  InitialConditionSource=Input port  SampleTime=filtDV.dT
      settings: InputPortMap=u0,p4
  Delay2 : Delay  DelayLength=0  InitialConditionSource=Input port  SampleTime=filtDV.dT
      settings: InputPortMap=u0,p4
  Delay3 : Delay  InitialConditionSource=Input port  SampleTime=filtDV.dT
      settings: InputPortMap=u0,p4
  Delay4 : Delay  DelayLength=1  InitialConditionSource=Input port  SampleTime=filtDV.dT
      settings: InputPortMap=u0,p4
  Gain : Gain  Gain=filtDV.a0
  Gain1 : Gain  Gain=filtDV.b1
  Gain2 : Gain  Gain=filtDV.b2
  Gain3 : Gain  Gain=filtDV.b0
  Gain4 : Gain  Gain=filtDV.a1
  Sum : Sum  Inputs=|--+++
  dVFilt : Outport
  wires:
  Gain3/1 -> Sum/5
  Gain2/1 -> Sum/3
  Delay4/1 -> Gain4/1
  Delay/1 -> Gain/1
  Delay1/1 -> Gain1/1
  Delay2/1 -> Gain2/1
  Gain4/1 -> Sum/1
  Sum/1 -> dVFilt/1, Delay4/1, Delay/1  "dVFilt"
  dV/1 -> Delay2/1, Delay2/2, Delay1/1, Delay3/2, Delay3/1, Delay1/2, Delay4/2, Delay/2  "dV"
  Gain1/1 -> Sum/4
  Gain/1 -> Sum/2
  Delay3/1 -> Gain3/1

== system SimForces2020a/sbVDCController/sbFormTotalRequiredForces/sbTotalRequiredForcesRS1/sbFilteredVelocityDerivativeB41/sbLowPassFilter4 ==
  dV : Inport
  Delay : Delay  InitialConditionSource=Input port  SampleTime=filtDV.dT
      settings: InputPortMap=u0,p4
  Delay1 : Delay  DelayLength=1  InitialConditionSource=Input port  SampleTime=filtDV.dT
      settings: InputPortMap=u0,p4
  Delay2 : Delay  DelayLength=0  InitialConditionSource=Input port  SampleTime=filtDV.dT
      settings: InputPortMap=u0,p4
  Delay3 : Delay  InitialConditionSource=Input port  SampleTime=filtDV.dT
      settings: InputPortMap=u0,p4
  Delay4 : Delay  DelayLength=1  InitialConditionSource=Input port  SampleTime=filtDV.dT
      settings: InputPortMap=u0,p4
  Gain : Gain  Gain=filtDV.a0
  Gain1 : Gain  Gain=filtDV.b1
  Gain2 : Gain  Gain=filtDV.b2
  Gain3 : Gain  Gain=filtDV.b0
  Gain4 : Gain  Gain=filtDV.a1
  Sum : Sum  Inputs=|--+++
  dVFilt : Outport
  wires:
  Delay3/1 -> Gain3/1
  Gain/1 -> Sum/2
  Gain1/1 -> Sum/4
  dV/1 -> Delay/2, Delay4/2, Delay1/2, Delay3/1, Delay3/2, Delay1/1, Delay2/2, Delay2/1  "dV"
  Sum/1 -> Delay/1, Delay4/1, dVFilt/1  "dVFilt"
  Gain4/1 -> Sum/1
  Delay2/1 -> Gain2/1
  Delay1/1 -> Gain1/1
  Delay/1 -> Gain/1
  Delay4/1 -> Gain4/1
  Gain2/1 -> Sum/3
  Gain3/1 -> Sum/5

== system SimForces2020a/sbVDCController/sbFormTotalRequiredForces/sbTotalRequiredForcesRS1/sbFilteredVelocityDerivativeB41/sbLowPassFilter5 ==
  dV : Inport
  Delay : Delay  InitialConditionSource=Input port  SampleTime=filtDV.dT
      settings: InputPortMap=u0,p4
  Delay1 : Delay  DelayLength=1  InitialConditionSource=Input port  SampleTime=filtDV.dT
      settings: InputPortMap=u0,p4
  Delay2 : Delay  DelayLength=0  InitialConditionSource=Input port  SampleTime=filtDV.dT
      settings: InputPortMap=u0,p4
  Delay3 : Delay  InitialConditionSource=Input port  SampleTime=filtDV.dT
      settings: InputPortMap=u0,p4
  Delay4 : Delay  DelayLength=1  InitialConditionSource=Input port  SampleTime=filtDV.dT
      settings: InputPortMap=u0,p4
  Gain : Gain  Gain=filtDV.a0
  Gain1 : Gain  Gain=filtDV.b1
  Gain2 : Gain  Gain=filtDV.b2
  Gain3 : Gain  Gain=filtDV.b0
  Gain4 : Gain  Gain=filtDV.a1
  Sum : Sum  Inputs=|--+++
  dVFilt : Outport
  wires:
  Gain3/1 -> Sum/5
  Gain2/1 -> Sum/3
  Delay4/1 -> Gain4/1
  Delay/1 -> Gain/1
  Delay1/1 -> Gain1/1
  Delay2/1 -> Gain2/1
  Gain4/1 -> Sum/1
  Sum/1 -> dVFilt/1, Delay4/1, Delay/1  "dVFilt"
  dV/1 -> Delay2/1, Delay2/2, Delay1/1, Delay3/2, Delay3/1, Delay1/2, Delay4/2, Delay/2  "dV"
  Gain1/1 -> Sum/4
  Gain/1 -> Sum/2
  Delay3/1 -> Gain3/1

== system SimForces2020a/sbVDCController/sbFormTotalRequiredForces/sbTotalRequiredForcesRS1/sbFilteredVelocityDerivativeB41/sbLowPassFilter6 ==
  dV : Inport
  Delay : Delay  InitialConditionSource=Input port  SampleTime=filtDV.dT
      settings: InputPortMap=u0,p4
  Delay1 : Delay  DelayLength=1  InitialConditionSource=Input port  SampleTime=filtDV.dT
      settings: InputPortMap=u0,p4
  Delay2 : Delay  DelayLength=0  InitialConditionSource=Input port  SampleTime=filtDV.dT
      settings: InputPortMap=u0,p4
  Delay3 : Delay  InitialConditionSource=Input port  SampleTime=filtDV.dT
      settings: InputPortMap=u0,p4
  Delay4 : Delay  DelayLength=1  InitialConditionSource=Input port  SampleTime=filtDV.dT
      settings: InputPortMap=u0,p4
  Gain : Gain  Gain=filtDV.a0
  Gain1 : Gain  Gain=filtDV.b1
  Gain2 : Gain  Gain=filtDV.b2
  Gain3 : Gain  Gain=filtDV.b0
  Gain4 : Gain  Gain=filtDV.a1
  Sum : Sum  Inputs=|--+++
  dVFilt : Outport
  wires:
  Delay3/1 -> Gain3/1
  Gain/1 -> Sum/2
  Gain1/1 -> Sum/4
  dV/1 -> Delay/2, Delay4/2, Delay1/2, Delay3/1, Delay3/2, Delay1/1, Delay2/2, Delay2/1  "dV"
  Sum/1 -> Delay/1, Delay4/1, dVFilt/1  "dVFilt"
  Gain4/1 -> Sum/1
  Delay2/1 -> Gain2/1
  Delay1/1 -> Gain1/1
  Delay/1 -> Gain/1
  Delay4/1 -> Gain4/1
  Gain2/1 -> Sum/3
  Gain3/1 -> Sum/5

== system SimForces2020a/sbVDCController/sbFormTotalRequiredForces/sbTotalRequiredForcesRS1/sbFilteredVelocityDerivativeBc1/sbDiscreteDerivative1 ==
  u : Inport
  Add : Sum  Inputs=-+
  Gain6 : Gain  Gain=1/(2*controller.dT)
  Integer Delay : Delay  InitialConditionSource=Input port  InitialCondition=0  SampleTime=controller.dT
      settings: InputPortMap=u0,p4
  du/dt : Outport  PortDimensions=1
  wires:
  Gain6/1 -> du/dt/1
  Integer Delay/1 -> Add/1
  u/1 -> Add/2, Integer Delay/2, Integer Delay/1
  Add/1 -> Gain6/1

== system SimForces2020a/sbVDCController/sbFormTotalRequiredForces/sbTotalRequiredForcesRS1/sbFilteredVelocityDerivativeBc1/sbDiscreteDerivative2 ==
  u : Inport
  Add : Sum  Inputs=-+
  Gain6 : Gain  Gain=1/(2*controller.dT)
  Integer Delay : Delay  InitialConditionSource=Input port  InitialCondition=0  SampleTime=controller.dT
      settings: InputPortMap=u0,p4
  du/dt : Outport  PortDimensions=1
  wires:
  Gain6/1 -> du/dt/1
  Add/1 -> Gain6/1
  Integer Delay/1 -> Add/1
  u/1 -> Add/2, Integer Delay/2, Integer Delay/1

== system SimForces2020a/sbVDCController/sbFormTotalRequiredForces/sbTotalRequiredForcesRS1/sbFilteredVelocityDerivativeBc1/sbDiscreteDerivative3 ==
  u : Inport
  Add : Sum  Inputs=-+
  Gain6 : Gain  Gain=1/(2*controller.dT)
  Integer Delay : Delay  InitialConditionSource=Input port  InitialCondition=0  SampleTime=controller.dT
      settings: InputPortMap=u0,p4
  du/dt : Outport  PortDimensions=1
  wires:
  Gain6/1 -> du/dt/1
  u/1 -> Add/2, Integer Delay/2, Integer Delay/1
  Integer Delay/1 -> Add/1
  Add/1 -> Gain6/1

== system SimForces2020a/sbVDCController/sbFormTotalRequiredForces/sbTotalRequiredForcesRS1/sbFilteredVelocityDerivativeBc1/sbDiscreteDerivative4 ==
  u : Inport
  Add : Sum  Inputs=-+
  Gain6 : Gain  Gain=1/(2*controller.dT)
  Integer Delay : Delay  InitialConditionSource=Input port  InitialCondition=0  SampleTime=controller.dT
      settings: InputPortMap=u0,p4
  du/dt : Outport  PortDimensions=1
  wires:
  Gain6/1 -> du/dt/1
  u/1 -> Add/2, Integer Delay/2, Integer Delay/1
  Integer Delay/1 -> Add/1
  Add/1 -> Gain6/1

== system SimForces2020a/sbVDCController/sbFormTotalRequiredForces/sbTotalRequiredForcesRS1/sbFilteredVelocityDerivativeBc1/sbDiscreteDerivative5 ==
  u : Inport
  Add : Sum  Inputs=-+
  Gain6 : Gain  Gain=1/(2*controller.dT)
  Integer Delay : Delay  InitialConditionSource=Input port  InitialCondition=0  SampleTime=controller.dT
      settings: InputPortMap=u0,p4
  du/dt : Outport  PortDimensions=1
  wires:
  Gain6/1 -> du/dt/1
  u/1 -> Add/2, Integer Delay/2, Integer Delay/1
  Integer Delay/1 -> Add/1
  Add/1 -> Gain6/1

== system SimForces2020a/sbVDCController/sbFormTotalRequiredForces/sbTotalRequiredForcesRS1/sbFilteredVelocityDerivativeBc1/sbDiscreteDerivative6 ==
  u : Inport
  Add : Sum  Inputs=-+
  Gain6 : Gain  Gain=1/(2*controller.dT)
  Integer Delay : Delay  InitialConditionSource=Input port  InitialCondition=0  SampleTime=controller.dT
      settings: InputPortMap=u0,p4
  du/dt : Outport  PortDimensions=1
  wires:
  Gain6/1 -> du/dt/1
  u/1 -> Add/2, Integer Delay/2, Integer Delay/1
  Integer Delay/1 -> Add/1
  Add/1 -> Gain6/1

== system SimForces2020a/sbVDCController/sbFormTotalRequiredForces/sbTotalRequiredForcesRS1/sbFilteredVelocityDerivativeBc1/sbLowPassFilter1 ==
  dV : Inport
  Delay : Delay  InitialConditionSource=Input port  SampleTime=filtDV.dT
      settings: InputPortMap=u0,p4
  Delay1 : Delay  DelayLength=1  InitialConditionSource=Input port  SampleTime=filtDV.dT
      settings: InputPortMap=u0,p4
  Delay2 : Delay  DelayLength=0  InitialConditionSource=Input port  SampleTime=filtDV.dT
      settings: InputPortMap=u0,p4
  Delay3 : Delay  InitialConditionSource=Input port  SampleTime=filtDV.dT
      settings: InputPortMap=u0,p4
  Delay4 : Delay  DelayLength=1  InitialConditionSource=Input port  SampleTime=filtDV.dT
      settings: InputPortMap=u0,p4
  Gain : Gain  Gain=filtDV.a0
  Gain1 : Gain  Gain=filtDV.b1
  Gain2 : Gain  Gain=filtDV.b2
  Gain3 : Gain  Gain=filtDV.b0
  Gain4 : Gain  Gain=filtDV.a1
  Sum : Sum  Inputs=|--+++
  dVFilt : Outport
  wires:
  Delay3/1 -> Gain3/1
  Gain/1 -> Sum/2
  Gain1/1 -> Sum/4
  dV/1 -> Delay/2, Delay4/2, Delay1/2, Delay3/1, Delay3/2, Delay1/1, Delay2/2, Delay2/1  "dV"
  Sum/1 -> Delay/1, Delay4/1, dVFilt/1  "dVFilt"
  Gain4/1 -> Sum/1
  Delay2/1 -> Gain2/1
  Delay1/1 -> Gain1/1
  Delay/1 -> Gain/1
  Delay4/1 -> Gain4/1
  Gain2/1 -> Sum/3
  Gain3/1 -> Sum/5

== system SimForces2020a/sbVDCController/sbFormTotalRequiredForces/sbTotalRequiredForcesRS1/sbFilteredVelocityDerivativeBc1/sbLowPassFilter2 ==
  dV : Inport
  Delay : Delay  InitialConditionSource=Input port  SampleTime=filtDV.dT
      settings: InputPortMap=u0,p4
  Delay1 : Delay  DelayLength=1  InitialConditionSource=Input port  SampleTime=filtDV.dT
      settings: InputPortMap=u0,p4
  Delay2 : Delay  DelayLength=0  InitialConditionSource=Input port  SampleTime=filtDV.dT
      settings: InputPortMap=u0,p4
  Delay3 : Delay  InitialConditionSource=Input port  SampleTime=filtDV.dT
      settings: InputPortMap=u0,p4
  Delay4 : Delay  DelayLength=1  InitialConditionSource=Input port  SampleTime=filtDV.dT
      settings: InputPortMap=u0,p4
  Gain : Gain  Gain=filtDV.a0
  Gain1 : Gain  Gain=filtDV.b1
  Gain2 : Gain  Gain=filtDV.b2
  Gain3 : Gain  Gain=filtDV.b0
  Gain4 : Gain  Gain=filtDV.a1
  Sum : Sum  Inputs=|--+++
  dVFilt : Outport
  wires:
  Gain3/1 -> Sum/5
  Gain2/1 -> Sum/3
  Delay4/1 -> Gain4/1
  Delay/1 -> Gain/1
  Delay1/1 -> Gain1/1
  Delay2/1 -> Gain2/1
  Gain4/1 -> Sum/1
  Sum/1 -> dVFilt/1, Delay4/1, Delay/1  "dVFilt"
  dV/1 -> Delay2/1, Delay2/2, Delay1/1, Delay3/2, Delay3/1, Delay1/2, Delay4/2, Delay/2  "dV"
  Gain1/1 -> Sum/4
  Gain/1 -> Sum/2
  Delay3/1 -> Gain3/1

== system SimForces2020a/sbVDCController/sbFormTotalRequiredForces/sbTotalRequiredForcesRS1/sbFilteredVelocityDerivativeBc1/sbLowPassFilter3 ==
  dV : Inport
  Delay : Delay  InitialConditionSource=Input port  SampleTime=filtDV.dT
      settings: InputPortMap=u0,p4
  Delay1 : Delay  DelayLength=1  InitialConditionSource=Input port  SampleTime=filtDV.dT
      settings: InputPortMap=u0,p4
  Delay2 : Delay  DelayLength=0  InitialConditionSource=Input port  SampleTime=filtDV.dT
      settings: InputPortMap=u0,p4
  Delay3 : Delay  InitialConditionSource=Input port  SampleTime=filtDV.dT
      settings: InputPortMap=u0,p4
  Delay4 : Delay  DelayLength=1  InitialConditionSource=Input port  SampleTime=filtDV.dT
      settings: InputPortMap=u0,p4
  Gain : Gain  Gain=filtDV.a0
  Gain1 : Gain  Gain=filtDV.b1
  Gain2 : Gain  Gain=filtDV.b2
  Gain3 : Gain  Gain=filtDV.b0
  Gain4 : Gain  Gain=filtDV.a1
  Sum : Sum  Inputs=|--+++
  dVFilt : Outport
  wires:
  Delay3/1 -> Gain3/1
  Gain/1 -> Sum/2
  Gain1/1 -> Sum/4
  dV/1 -> Delay/2, Delay4/2, Delay1/2, Delay3/1, Delay3/2, Delay1/1, Delay2/2, Delay2/1  "dV"
  Sum/1 -> Delay/1, Delay4/1, dVFilt/1  "dVFilt"
  Gain4/1 -> Sum/1
  Delay2/1 -> Gain2/1
  Delay1/1 -> Gain1/1
  Delay/1 -> Gain/1
  Delay4/1 -> Gain4/1
  Gain2/1 -> Sum/3
  Gain3/1 -> Sum/5

== system SimForces2020a/sbVDCController/sbFormTotalRequiredForces/sbTotalRequiredForcesRS1/sbFilteredVelocityDerivativeBc1/sbLowPassFilter4 ==
  dV : Inport
  Delay : Delay  InitialConditionSource=Input port  SampleTime=filtDV.dT
      settings: InputPortMap=u0,p4
  Delay1 : Delay  DelayLength=1  InitialConditionSource=Input port  SampleTime=filtDV.dT
      settings: InputPortMap=u0,p4
  Delay2 : Delay  DelayLength=0  InitialConditionSource=Input port  SampleTime=filtDV.dT
      settings: InputPortMap=u0,p4
  Delay3 : Delay  InitialConditionSource=Input port  SampleTime=filtDV.dT
      settings: InputPortMap=u0,p4
  Delay4 : Delay  DelayLength=1  InitialConditionSource=Input port  SampleTime=filtDV.dT
      settings: InputPortMap=u0,p4
  Gain : Gain  Gain=filtDV.a0
  Gain1 : Gain  Gain=filtDV.b1
  Gain2 : Gain  Gain=filtDV.b2
  Gain3 : Gain  Gain=filtDV.b0
  Gain4 : Gain  Gain=filtDV.a1
  Sum : Sum  Inputs=|--+++
  dVFilt : Outport
  wires:
  Gain3/1 -> Sum/5
  Gain2/1 -> Sum/3
  Delay4/1 -> Gain4/1
  Delay/1 -> Gain/1
  Delay1/1 -> Gain1/1
  Delay2/1 -> Gain2/1
  Gain4/1 -> Sum/1
  Sum/1 -> dVFilt/1, Delay4/1, Delay/1  "dVFilt"
  dV/1 -> Delay2/1, Delay2/2, Delay1/1, Delay3/2, Delay3/1, Delay1/2, Delay4/2, Delay/2  "dV"
  Gain1/1 -> Sum/4
  Gain/1 -> Sum/2
  Delay3/1 -> Gain3/1

== system SimForces2020a/sbVDCController/sbFormTotalRequiredForces/sbTotalRequiredForcesRS1/sbFilteredVelocityDerivativeBc1/sbLowPassFilter5 ==
  dV : Inport
  Delay : Delay  InitialConditionSource=Input port  SampleTime=filtDV.dT
      settings: InputPortMap=u0,p4
  Delay1 : Delay  DelayLength=1  InitialConditionSource=Input port  SampleTime=filtDV.dT
      settings: InputPortMap=u0,p4
  Delay2 : Delay  DelayLength=0  InitialConditionSource=Input port  SampleTime=filtDV.dT
      settings: InputPortMap=u0,p4
  Delay3 : Delay  InitialConditionSource=Input port  SampleTime=filtDV.dT
      settings: InputPortMap=u0,p4
  Delay4 : Delay  DelayLength=1  InitialConditionSource=Input port  SampleTime=filtDV.dT
      settings: InputPortMap=u0,p4
  Gain : Gain  Gain=filtDV.a0
  Gain1 : Gain  Gain=filtDV.b1
  Gain2 : Gain  Gain=filtDV.b2
  Gain3 : Gain  Gain=filtDV.b0
  Gain4 : Gain  Gain=filtDV.a1
  Sum : Sum  Inputs=|--+++
  dVFilt : Outport
  wires:
  Delay3/1 -> Gain3/1
  Gain/1 -> Sum/2
  Gain1/1 -> Sum/4
  dV/1 -> Delay/2, Delay4/2, Delay1/2, Delay3/1, Delay3/2, Delay1/1, Delay2/2, Delay2/1  "dV"
  Sum/1 -> Delay/1, Delay4/1, dVFilt/1  "dVFilt"
  Gain4/1 -> Sum/1
  Delay2/1 -> Gain2/1
  Delay1/1 -> Gain1/1
  Delay/1 -> Gain/1
  Delay4/1 -> Gain4/1
  Gain2/1 -> Sum/3
  Gain3/1 -> Sum/5

== system SimForces2020a/sbVDCController/sbFormTotalRequiredForces/sbTotalRequiredForcesRS1/sbFilteredVelocityDerivativeBc1/sbLowPassFilter6 ==
  dV : Inport
  Delay : Delay  InitialConditionSource=Input port  SampleTime=filtDV.dT
      settings: InputPortMap=u0,p4
  Delay1 : Delay  DelayLength=1  InitialConditionSource=Input port  SampleTime=filtDV.dT
      settings: InputPortMap=u0,p4
  Delay2 : Delay  DelayLength=0  InitialConditionSource=Input port  SampleTime=filtDV.dT
      settings: InputPortMap=u0,p4
  Delay3 : Delay  InitialConditionSource=Input port  SampleTime=filtDV.dT
      settings: InputPortMap=u0,p4
  Delay4 : Delay  DelayLength=1  InitialConditionSource=Input port  SampleTime=filtDV.dT
      settings: InputPortMap=u0,p4
  Gain : Gain  Gain=filtDV.a0
  Gain1 : Gain  Gain=filtDV.b1
  Gain2 : Gain  Gain=filtDV.b2
  Gain3 : Gain  Gain=filtDV.b0
  Gain4 : Gain  Gain=filtDV.a1
  Sum : Sum  Inputs=|--+++
  dVFilt : Outport
  wires:
  Gain3/1 -> Sum/5
  Gain2/1 -> Sum/3
  Delay4/1 -> Gain4/1
  Delay/1 -> Gain/1
  Delay1/1 -> Gain1/1
  Delay2/1 -> Gain2/1
  Gain4/1 -> Sum/1
  Sum/1 -> dVFilt/1, Delay4/1, Delay/1  "dVFilt"
  dV/1 -> Delay2/1, Delay2/2, Delay1/1, Delay3/2, Delay3/1, Delay1/2, Delay4/2, Delay/2  "dV"
  Gain1/1 -> Sum/4
  Gain/1 -> Sum/2
  Delay3/1 -> Gain3/1

== system SimForces2020a/sbVDCController/sbFormTotalRequiredForces/sbTotalRequiredForcesRS2/sbFilteredVelocityDerivativeB12/sbDiscreteDerivative1 ==
  u : Inport
  Add : Sum  Inputs=-+
  Gain6 : Gain  Gain=1/(2*controller.dT)
  Integer Delay : Delay  InitialConditionSource=Input port  InitialCondition=0  SampleTime=controller.dT
      settings: InputPortMap=u0,p4
  du/dt : Outport  PortDimensions=1
  wires:
  Add/1 -> Gain6/1
  u/1 -> Integer Delay/1, Integer Delay/2, Add/2
  Integer Delay/1 -> Add/1
  Gain6/1 -> du/dt/1
